simulink model "oog_example"  (R2016a)
settings: Solver=ode5  SolverMode=SingleTasking  StartTime=0.0  StopTime=Ttot  FixedStep=min(Ts_phy,Ts_sim)  RelTol=1e-3
PreLoadFcn:
  | oog_example_init
InitFcn:
  | oog_example_init
values from neighbouring files (symbols this model uses):
  col = {}    [oog_example_init.m]
  flex = {}    [oog_example_init.m]
  systemBase = {}    [oog_example_init.m]
  Ts = Ts_c    (= 0.0001)    [oog_example_init.m]
  Ts_phy = 1*Ts_sim    (= 0.0001)    [oog_example_init.m]
  Ts_sim = 100e-6    (= 0.0001)    [oog_example_init.m]
  wt1 = {}    [oog_example_init.m]
  wt2 = wt1    [oog_example_init.m]
  wt3 = wt1    [oog_example_init.m]
undefined symbols (not defined in the file or in its folder): avr, D1, Delta, DiscIntNeverNeededParam, governor, interface, Lf1, sm
libraries: powerlib x49, simulink_extras x35, pwrsysBasic x30, powerlib_meascontrol x17, pwrsysVICtrl x15, simulink x5, pwrsysVSrc x4, pwrsysTransf x4
(part 1 of 3)
settings Model: Creator=Freya_super  LastModifiedBy=ericfa
settings DataIOCC: LimitDataPoints=on  SaveFormat=Array  SaveOutput=off  SaveTime=off
settings OptimizationCC: BlockReduction=off  OptimizeBlockIOStorage=off  BufferReuse=off  GlobalBufferReuse=off  ExpressionFolding=off  LocalBlockOutputs=off
settings DebuggingCC: SolverPrmCheckMsg=warning  StateNameClashWarn=warning
settings HardwareCC: ProdBitPerPointer=32  ProdLargestAtomicFloat=None  ProdIntDivRoundTo=Undefined  ProdEndianess=Unspecified  ProdWordSize=32  ProdHWDeviceType=32-bit Generic
settings ModelReferenceCC: PropagateSignalLabelsOutOfModel=off
settings RTWCC: SystemTargetFile=rtlab_rtmodel.tlc  TemplateMakefile=rtlab_rtmodel.tmf  Description=RT-LAB Real-Time Target for Windows, and OPAL-RT Linux.
settings GRTTargetCC: GeneratePreprocessorConditionals=Use local settings  UseToolchainInfoCompliant=off
settings ConfigComp: CovModelRefEnable=Off

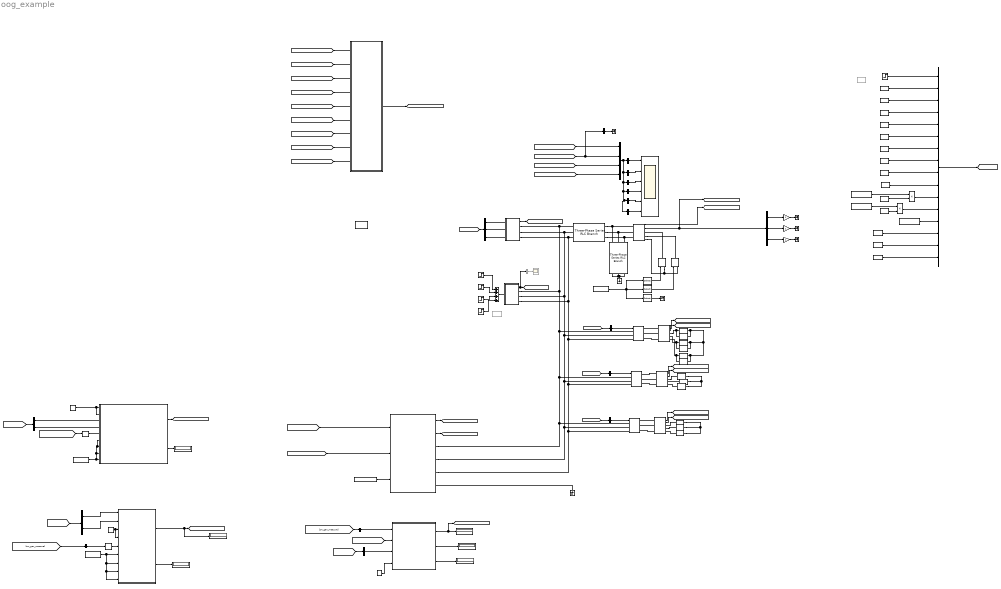
== system oog_example ==
  note: Egston terminals
  note: RMS and power calculation
  note: Automatic voltage regulator
  note: Back emf + reactance
  note: Mech.rotation
  note: Governor
  note: SM Generator (simple model)
  note: Load 3
  note: Load 2
  note: Load 1
  note: Commands
  note: Wind
      | farm
  Active : BusSelector  OutputSignals=genMeas.Pgen_pu,flexMeas.Pavg_pu,wfMeas.WT1.Pavg_pu,wfMeas.WT2.Pavg_pu,wfMeas.WT3.Pavg_pu  OutputAsBus=on
  Automatic voltage regulator : Subsystem
  Bus Creator1 : BusCreator  Inputs=4
  Bus Creator9 : BusCreator  Inputs=16
  Bus Selector1 : BusSelector  OutputSignals=load1_connect
  Bus Selector10 : BusSelector  OutputSignals=sm_backEmfPowerMeasure_pu
  Bus Selector11 : BusSelector  OutputSignals=load2_connect
  Bus Selector12 : BusSelector  OutputSignals=load3_connect
  Bus Selector4 : BusSelector  OutputSignals=freqReference pu,deltaFreqRef pu
  Bus Selector6 : BusSelector  OutputSignals=voltRef_WT1_pu,voltRef_WT2_pu,voltRef_WT3_pu
  Bus Selector7 : BusSelector  OutputSignals=freqReference pu
  Bus Selector8 : BusSelector  OutputSignals=voltRef_GT_pu,deltaVoltRef pu
  Bus Selector9 : BusSelector  OutputSignals=Vgen_filt [pu]
  Constant1 : Constant  Value=sm.phaseInitial  SampleTime=-1
  Constant{4..5,7,10,12} (5 alike) : Constant  Value=0  SampleTime=-1
  Constant13 : Constant  Commented=on  Value=0  SampleTime=Ts_sim
  Constant6 : Constant  Value=[0 0 0]  SampleTime=-1
  DC currents : BusSelector  OutputSignals=flexMeas.Idc_pu,wfMeas.WT1.Idc_pu,wfMeas.WT2.Idc_pu,wfMeas.WT3.Idc_pu  OutputAsBus=on
  DC voltages : BusSelector  OutputSignals=flexMeas.Vdc_pu,wfMeas.WT1.Vdc_pu,wfMeas.WT2.Vdc_pu,wfMeas.WT3.Vdc_pu  OutputAsBus=on
  Demux1 : Demux  Outputs=3
  Display{,1..5} (6 alike) : Display
  Flex : Subsystem
  Frequency : BusSelector  OutputSignals=genMeas.sm_freq [pu]
  Gain1 : Gain
  Gain2 : Gain
  Gain3 : Gain
  Ground1 : powerlib/Elements/Ground  LConnTagsString=a
  Ground3 : powerlib/Elements/Ground  LConnTagsString=a
  IL : powerlib/Electrical Sources/Controlled Current Source  Initialize=on  Source_Type=AC  Amplitude=0  Phase=0  Frequency=0  Measurements=None
  IL1 : powerlib/Electrical Sources/Controlled Current Source  Initialize=on  Source_Type=AC  Amplitude=0  Phase=0  Frequency=0  Measurements=None
  Memory1 : Memory
  Memory2 : Memory
  RL1 : powerlib/Elements/Series RLC Branch  LConnTagsString=__new0  RConnTagsString=__new0  BranchType=R  Resistance=load.R(1)  Inductance=load.L(1)  SetiL0=off  InitialCurrent=0  Capacitance=1e-6  Setx0=off  InitialVoltage=0  Measurements=None
  RL10 : powerlib/Elements/Series RLC Branch  LConnTagsString=__new0  RConnTagsString=__new0  BranchType=L  Resistance=load.R(1)  Inductance=load.L(1)  SetiL0=off  InitialCurrent=0  Capacitance=1e-6  Setx0=off  InitialVoltage=0  Measurements=None
  RL11 : powerlib/Elements/Series RLC Branch  LConnTagsString=__new0  RConnTagsString=__new0  BranchType=R  Resistance=load.R(1)  Inductance=load.L(1)  SetiL0=off  InitialCurrent=0  Capacitance=1e-6  Setx0=off  InitialVoltage=0  Measurements=None
  RL12 : powerlib/Elements/Series RLC Branch  LConnTagsString=__new0  RConnTagsString=__new0  BranchType=L  Resistance=load.R(1)  Inductance=load.L(1)  SetiL0=off  InitialCurrent=0  Capacitance=1e-6  Setx0=off  InitialVoltage=0  Measurements=None
  RL2 : powerlib/Elements/Series RLC Branch  LConnTagsString=__new0  RConnTagsString=__new0  BranchType=R  Resistance=load.R(1)  Inductance=load.L(1)  SetiL0=off  InitialCurrent=0  Capacitance=1e-6  Setx0=off  InitialVoltage=0  Measurements=None
  RL3 : powerlib/Elements/Series RLC Branch  LConnTagsString=__new0  RConnTagsString=__new0  BranchType=L  Resistance=load.R(1)  Inductance=load.L(1)  SetiL0=off  InitialCurrent=0  Capacitance=1e-6  Setx0=off  InitialVoltage=0  Measurements=None
  RL4 : powerlib/Elements/Series RLC Branch  LConnTagsString=__new0  RConnTagsString=__new0  BranchType=RL  Resistance=load.R(2)  Inductance=load.L(2)  SetiL0=off  InitialCurrent=0  Capacitance=1e-6  Setx0=off  InitialVoltage=0  Measurements=None
  RL5 : powerlib/Elements/Series RLC Branch  LConnTagsString=__new0  RConnTagsString=__new0  BranchType=RL  Resistance=load.R(2)  Inductance=load.L(2)  SetiL0=off  InitialCurrent=0  Capacitance=1e-6  Setx0=off  InitialVoltage=0  Measurements=None
  RL6 : powerlib/Elements/Series RLC Branch  LConnTagsString=__new0  RConnTagsString=__new0  BranchType=RL  Resistance=load.R(2)  Inductance=load.L(2)  SetiL0=off  InitialCurrent=0  Capacitance=1e-6  Setx0=off  InitialVoltage=0  Measurements=None
  RL7 : powerlib/Elements/Series RLC Branch  LConnTagsString=__new0  RConnTagsString=__new0  BranchType=RL  Resistance=load.R(3)  Inductance=load.L(3)  SetiL0=off  InitialCurrent=0  Capacitance=1e-6  Setx0=off  InitialVoltage=0  Measurements=None
  RL8 : powerlib/Elements/Series RLC Branch  LConnTagsString=__new0  RConnTagsString=__new0  BranchType=RL  Resistance=load.R(3)  Inductance=load.L(3)  SetiL0=off  InitialCurrent=0  Capacitance=1e-6  Setx0=off  InitialVoltage=0  Measurements=None
  RL9 : powerlib/Elements/Series RLC Branch  LConnTagsString=__new0  RConnTagsString=__new0  BranchType=RL  Resistance=load.R(3)  Inductance=load.L(3)  SetiL0=off  InitialCurrent=0  Capacitance=1e-6  Setx0=off  InitialVoltage=0  Measurements=None
  Reactive : BusSelector  OutputSignals=genMeas.Qgen_pu,flexMeas.Qavg_pu,wfMeas.WT1.Qavg_pu,wfMeas.WT2.Qavg_pu,wfMeas.WT3.Qavg_pu  OutputAsBus=on
  Rotation1 : Subsystem
  SM_simple : Subsystem
  Scope_All : Scope  NumInputPorts=6
  Scope_Flex : Scope  Commented=on
  Selector6 : Selector  InputPortWidth=3  IndexOptions=Index vector (dialog)  Indices=[1]  OutputSizes=1
  Selector7 : Selector  InputPortWidth=3  IndexOptions=Index vector (dialog)  Indices=2  OutputSizes=1
  Selector8 : Selector  InputPortWidth=3  IndexOptions=Index vector (dialog)  Indices=3  OutputSizes=1
  Step : Step  Time=3  SampleTime=0
  Step1 : Step  Time=7  After=-0.2  SampleTime=0
  Step2 : Step  Time=7.5  After=-0.2  SampleTime=0
  Step3 : Step  Time=8  After=-0.2  SampleTime=0
  Step4 : Step  Time=8.5  After=-0.2  SampleTime=0
  Sum : Sum  Inputs=4
  Terminator{,1..4} (5 alike) : Terminator
  Three-Phase Series RLC Branch : powerlib/Elements/Three-Phase Series RLC Branch  LConnTagsString=A|B|C  RConnTagsString=A|B|C  BranchType=R  Resistance=interface.Rs  Inductance=1e-3  Capacitance=1e-6  Measurements=None
  Three-Phase Series RLC Branch1 : powerlib/Elements/Three-Phase Series RLC Branch  LConnTagsString=A|B|C  RConnTagsString=A|B|C  BranchType=R  Resistance=interface.Rp  Inductance=1e-3  Capacitance=1e-6  Measurements=None
  Three-Phase V-I Measurement{,1..3} (4 alike) : powerlib/Measurements/Three-Phase V-I Measurement  VoltageMeasurement=phase-to-ground  SetLabelV=off  LabelV=Vabc  Vpu=off  VpuLL=off  CurrentMeasurement=yes  SetLabelI=off  LabelI=Iabc  Ipu=off  Pbase=100e6  Vbase=500e3  OutputType=Complex  PhasorSimulation=off  PSBequivalent=0
  Three-Phase Breaker : powerlib/Elements/Three-Phase Breaker  InitialState=open  SwitchA=on  SwitchB=on  SwitchC=on  SwitchTimes="[4/60  10/60]"  External=on  BreakerResistance=0.001  SnubberResistance=1e6  SnubberCapacitance=inf  Measurements=None
  Three-Phase Breaker1 : powerlib/Elements/Three-Phase Breaker  InitialState=open  SwitchA=on  SwitchB=on  SwitchC=on  SwitchTimes="[4/60  10/60]"  External=on  BreakerResistance=0.001  SnubberResistance=1e6  SnubberCapacitance=inf  Measurements=None
  Three-Phase Breaker2 : powerlib/Elements/Three-Phase Breaker  InitialState=open  SwitchA=on  SwitchB=on  SwitchC=on  SwitchTimes="[4/60  10/60]"  External=on  BreakerResistance=0.001  SnubberResistance=1e6  SnubberCapacitance=inf  Measurements=None
  Trigger_Data_Logging : Constant  Value=0  SampleTime=-1
  Turbine Governor1 : Subsystem
  Voltage : BusSelector  OutputSignals=genMeas.Vgen_filt [pu],flexMeas.Vavg_pu,wfMeas.WT1.Vavg_pu,wfMeas.WT2.Vavg_pu,wfMeas.WT3.Vavg_pu  OutputAsBus=on
  Wind Farm : Subsystem
  current_gain : Constant  Value=0.1  SampleTime=-1
  deltaFreqRef pu : Constant  Value=0  OutDataTypeStr=double  SampleTime=Ts
  deltaVoltRef pu : Constant  Value=0  OutDataTypeStr=double  SampleTime=Ts
  dfreqRefESS : Constant  Value=0  OutDataTypeStr=double  SampleTime=Ts
  dfreqRefGT : Constant  Value=0  OutDataTypeStr=double  SampleTime=Ts
  enableCurrentFeedback : Constant  Value=0  OutDataTypeStr=double  SampleTime=Ts
  enableVoltageOutput : Constant  Value=0  OutDataTypeStr=double  SampleTime=Ts
  flex : BusSelector  Commented=on  OutputSignals=Pavg_pu,Qavg_pu,Vavg_pu,Vdc_pu,Idc_pu  OutputAsBus=on
  freqReference pu : Constant  OutDataTypeStr=double  SampleTime=Ts
  gen : BusSelector  OutputSignals=Pgen_pu,Qgen_pu,Vgen_filt [pu]  OutputAsBus=on
  load1_connect : Constant  Commented=on  Value=0  OutDataTypeStr=double  SampleTime=Ts
  load2_connect : Constant  Value=0  OutDataTypeStr=double  SampleTime=Ts
  load3_connect : Constant  Value=0  OutDataTypeStr=double  SampleTime=Ts
  mul : Product  Inputs=**
  mul1 : Product  Inputs=**
  powergui : powerlib/powergui  Priority=1  SimulationMode=Discrete  SolverType=Tustin  SampleTime=max(Ts_phy,Ts_sim)  frequency=60  SPID=off  DisableSnubberDevices=off  DisableRonSwitches=off  DisableVfSwitches=off  SwTol=0  DisplayEquations=off  Interpol=off  ExternalGateDelay=off  methode=off  Ts=0  FunctionMessages=off  echomessages=off  HookPort=off  EnableUseOfTLC=off  x0status=blocks  frequencyindice=0  Pbase=100e6  ErrMax=1e-4  Iterations=50  UnitsV=kV  UnitsW=MW  buscounter=0  RestoreLinks=warning  ResistiveCurrentMeasurement=off  Frange=[0:2:500]  Ylog=off  Xlog=on  ShowGrid=off  save=off  variable=ZData  structure=0  ZoomFFT=off  StartTime=0.0  cycles=1  DisplayStyle=1  fundamental=60  FreqAxis=off  MaxFrequency=1000  frequencyindicesteady=1  RmsSteady=1  display=off
  rms and power calc : Subsystem
  voltRefESS : Constant  OutDataTypeStr=double  SampleTime=Ts
  voltRefGT : Constant  OutDataTypeStr=double  SampleTime=Ts
  voltRefWT1 : Constant  OutDataTypeStr=double  SampleTime=Ts
  voltRefWT2 : Constant  OutDataTypeStr=double  SampleTime=Ts
  voltRefWT3 : Constant  OutDataTypeStr=double  SampleTime=Ts
  voltage_gain : Constant  Value=0.1  SampleTime=-1
  wires:
  Bus Selector12/1 -> Three-Phase Breaker2/1  "<load3_connect>"
  [fromGUI] -> Bus Selector12/1
  Bus Selector11/1 -> Three-Phase Breaker1/1  "<load2_connect>"
  [fromGUI] -> Bus Selector11/1
  Bus Selector1/1 -> Three-Phase Breaker/1  "<load1_connect>"
  [fromGUI] -> Bus Selector1/1
  Three-Phase V-I Measurement2/1 -> [V_abc_L3]
  Three-Phase V-I Measurement2/2 -> [I_abc_L3]
  Three-Phase V-I Measurement1/1 -> [V_abc_L2]
  Three-Phase V-I Measurement1/2 -> [I_abc_L2]
  Three-Phase V-I Measurement3/2 -> [I_abc_L1]
  Three-Phase V-I Measurement3/1 -> [V_abc_L1]
  Bus Selector10/1 -> Rotation1/1(generator power (pu))  "<sm_backEmfPowerMeasure_pu>"
  [sm_gen_measure] -> Bus Selector10/1
  Bus Selector9/1 -> Memory2/1  "<Vgen_filt [pu]>"
  SM_simple/1(wt1) -> [wt]
  Memory2/1 -> Automatic voltage regulator/5(voltage_feedback (pu))
  Constant7/1 -> Rotation1/4(resetSpeed)
  Constant12/1 -> Automatic voltage regulator/6(qGen (pu)), Automatic voltage regulator/7(qRefDroop (pu)), Automatic voltage regulator/8(pGen (pu)), Automatic voltage regulator/9(pRefDroop (pu))
  Constant4/1 -> Automatic voltage regulator/4(Reset_integrator), Automatic voltage regulator/3(Reset_value)
  Bus Selector8/2 -> Automatic voltage regulator/2(deltaVoltageRef (pu))  "<deltaVoltRef pu>"
  Constant10/1 -> Turbine Governor1/9(pGen (pu)), Turbine Governor1/8(powerControlEnable), Turbine Governor1/7(pRef (pu)), Turbine Governor1/6(pRefDroop (pu))
  Bus Selector4/2 -> Turbine Governor1/4(deltaSpeedRef (pu))  "<deltaFreqRef pu>"
  Bus Selector4/1 -> Turbine Governor1/3(Speed_ref (pu))  "<freqReference pu>"
  Constant5/1 -> Turbine Governor1/2(Reset_value), Turbine Governor1/1(Reset_gov)  "<resetSpeedGov>"
  Bus Selector8/1 -> Automatic voltage regulator/1(Voltage_ref (pu))  "<voltRef_GT_pu>"
  [fromGUI] -> Bus Selector8/1
  Bus Selector7/1 -> Rotation1/3(InitialSpeed)  "<freqReference pu>"
  [fromGUI] -> Bus Selector7/1
  [fromGUI] -> Bus Selector4/1
  [drivingTorque_pu] -> Rotation1/2(driving torque (pu))
  Turbine Governor1/1(output (pu)) -> [drivingTorque_pu]
  [sm_gen_measure] -> Bus Selector9/1
  Automatic voltage regulator/2(voltageRefActual (pu)) -> Display5/1
  Automatic voltage regulator/1(output (pu)) -> Display3/1, [sm_dynamicVoltage_pu]
  Turbine Governor1/2(speedRefActual (pu)) -> Display4/1
  Memory1/1 -> Turbine Governor1/5(Speed_feedback (pu))
  [sm_dynamicSpeed_pu] -> Memory1/1
  Rotation1/3(electric torque (pu)) -> Display2/1
  Rotation1/2(mechanical torque (pu)) -> Display1/1
  Rotation1/1(turbine speed (pu)) -> Display/1, [sm_dynamicSpeed_pu]
  [sm_dynamicVoltage_pu] -> SM_simple/2(GenBackEmf [pu])
  SM_simple/2(sm_gen_measure) -> [sm_gen_measure]
  Constant1/1 -> SM_simple/3(Phase [rad])
  [sm_dynamicSpeed_pu] -> SM_simple/1(Frequency [pu])  "sm_freq"
  Gain3/1 -> Terminator3/1  "Ic"
  Demux1/3 -> Gain3/1
  Gain2/1 -> Terminator2/1  "Ib"
  Demux1/2 -> Gain2/1
  Gain1/1 -> Terminator1/1  "Ia"
  Demux1/1 -> Gain1/1
  Selector7/1 -> IL1/1
  Three-Phase V-I Measurement/2 -> Demux1/1, [I_abc_interface]  "I_abc"
  Selector8/1 -> Terminator/1
  Constant6/1 -> Selector6/1, Selector7/1, Selector8/1
  Three-Phase V-I Measurement/1 -> [V_abc_interface]  "V_abc"
  Selector6/1 -> IL/1
  [wt] -> rms and power calc/1(wt)
  [V_abc_L1] -> rms and power calc/2(L1_Vabc)
  [I_abc_L1] -> rms and power calc/3(L1_Iabc)
  [V_abc_L2] -> rms and power calc/4(L2_Vabc)
  [I_abc_L2] -> rms and power calc/5(L2_Iabc)
  [V_abc_L3] -> rms and power calc/6(L3_Vabc)
  [I_abc_L3] -> rms and power calc/7(L3_Iabc)
  [V_abc_interface] -> rms and power calc/8(Interface_Vabc)
  [I_abc_interface] -> rms and power calc/9(Interface_Iabc)
  rms and power calc/1(Out1) -> [electricModel_meas]
  deltaVoltRef pu/1 -> Bus Creator9/15  "deltaVoltRef pu"
  dfreqRefGT/1 -> Bus Creator9/9  "dfreqRef_GT_pu"
  deltaFreqRef pu/1 -> Bus Creator9/14  "deltaFreqRef pu"
  dfreqRefESS/1 -> Bus Creator9/10  "dfreqRef_ESS_pu"
  voltage_gain/1 -> mul1/1  "voltage_gain_grid_side"
  mul1/1 -> Bus Creator9/12  "voltage_gain_grid_side"
  voltRefESS/1 -> Bus Creator9/5  "voltRef_ESS_pu"
  voltRefWT1/1 -> Bus Creator9/6  "voltRef_WT1_pu"
  current_gain/1 -> mul/1  "PHIL_gain_grid_side"
  Bus Creator9/1 -> [fromGUI]  "fromGUI"
  voltRefWT3/1 -> Bus Creator9/8  "voltRef_WT3_pu"
  Trigger_Data_Logging/1 -> Bus Creator9/13  "enable_logging"
  load2_connect/1 -> Bus Creator9/2  "load2_connect"
  mul/1 -> Bus Creator9/11  "PHIL_gain_grid_side"
  voltRefWT2/1 -> Bus Creator9/7  "voltRef_WT2_pu"
  enableCurrentFeedback/1 -> mul/2
  Step/1 -> Bus Creator9/1  "load1_connect"
  load3_connect/1 -> Bus Creator9/3  "load3_connect"
  enableVoltageOutput/1 -> mul1/2
  voltRefGT/1 -> Bus Creator9/4  "voltRef_GT_pu"
  [wf_measure] -> Bus Creator1/4  "wfMeas"
  [electricModel_meas] -> Bus Creator1/1  "electricModel_meas"
  [sm_gen_measure] -> gen/1, Bus Creator1/2  "genMeas"
  [flex_measure] -> Bus Creator1/3  "flexMeas"
  freqReference pu/1 -> Bus Creator9/16  "freqReference pu"
  Voltage/1 -> Scope_All/1
  Reactive/1 -> Scope_All/2
  Frequency/1 -> Scope_All/3  "<sm_freq [pu]>"
  Active/1 -> Scope_All/4
  Wind Farm/1(m) -> [wf_measure]  "WF"
  Bus Selector6/2 -> Wind Farm/2(WT2_Vsp)  "<voltRef_WT2_pu>"
  Bus Selector6/3 -> Wind Farm/3(WT1_Vsp)  "<voltRef_WT3_pu>"
  Bus Selector6/1 -> Wind Farm/1(WT3_Vsp)  "<voltRef_WT1_pu>"
  [fromGUI] -> Bus Selector6/1
  Bus Creator1/1 -> Voltage/1, Reactive/1, DC currents/1, DC voltages/1, Active/1, Frequency/1
  Flex/1(m) -> flex/1, [flex_measure]
  flex/1 -> Scope_Flex/1
  Sum/1 -> Flex/1(Psp)
  Step1/1 -> Sum/1
  Step2/1 -> Sum/2
  Step3/1 -> Sum/3
  gen/1 -> Terminator4/1
  DC voltages/1 -> Scope_All/5
  DC currents/1 -> Scope_All/6
  Step4/1 -> Sum/4
  connections:
  RL9/RConn1 -- RL7/RConn1 -- RL8/RConn1
  RL4/RConn1 -- RL5/RConn1 -- RL6/RConn1
  RL1/RConn1 -- RL10/RConn1 -- RL12/RConn1 -- RL11/RConn1 -- RL3/RConn1 -- RL2/RConn1
  Three-Phase Breaker/LConn3 -- Three-Phase Breaker1/LConn3 -- Three-Phase Breaker2/LConn3 -- SM_simple/RConn3 -- Flex/RConn3 -- Wind Farm/RConn3 -- Three-Phase Series RLC Branch/LConn3
  Three-Phase Series RLC Branch/RConn1 -- Three-Phase V-I Measurement/LConn1 -- Three-Phase Series RLC Branch1/RConn1
  Three-Phase Series RLC Branch/RConn2 -- Three-Phase V-I Measurement/LConn2 -- Three-Phase Series RLC Branch1/RConn2
  Three-Phase Series RLC Branch/RConn3 -- Three-Phase V-I Measurement/LConn3 -- Three-Phase Series RLC Branch1/RConn3
  Three-Phase Series RLC Branch1/LConn1 -- Three-Phase Series RLC Branch1/LConn3 -- Ground1/LConn1 -- Three-Phase Series RLC Branch1/LConn2
  IL/LConn1 -- Three-Phase V-I Measurement/RConn3 -- IL1/LConn1
  Three-Phase V-I Measurement3/LConn1 -- Three-Phase Breaker/RConn1
  Three-Phase V-I Measurement3/RConn1 -- RL10/LConn1 -- RL1/LConn1
  Three-Phase V-I Measurement2/LConn3 -- Three-Phase Breaker2/RConn3
  Ground3/LConn1 -- SM_simple/RConn4
  Three-Phase V-I Measurement2/RConn2 -- RL9/LConn1
  Three-Phase V-I Measurement3/LConn2 -- Three-Phase Breaker/RConn2
  Three-Phase V-I Measurement1/LConn1 -- Three-Phase Breaker1/RConn1
  RL7/LConn1 -- Three-Phase V-I Measurement2/RConn3
  RL6/LConn1 -- Three-Phase V-I Measurement1/RConn3
  Three-Phase V-I Measurement1/RConn1 -- RL4/LConn1
  RL8/LConn1 -- Three-Phase V-I Measurement2/RConn1
  Three-Phase V-I Measurement2/LConn2 -- Three-Phase Breaker2/RConn2
  Three-Phase V-I Measurement1/LConn2 -- Three-Phase Breaker1/RConn2
  RL11/LConn1 -- RL12/LConn1 -- Three-Phase V-I Measurement3/RConn3
  Three-Phase V-I Measurement1/LConn3 -- Three-Phase Breaker1/RConn3
  Three-Phase V-I Measurement/RConn2 -- IL1/RConn1
  Three-Phase V-I Measurement2/LConn1 -- Three-Phase Breaker2/RConn1
  IL/RConn1 -- Three-Phase V-I Measurement/RConn1
  Three-Phase V-I Measurement3/LConn3 -- Three-Phase Breaker/RConn3
  RL2/LConn1 -- RL3/LConn1 -- Three-Phase V-I Measurement3/RConn2
  RL5/LConn1 -- Three-Phase V-I Measurement1/RConn2
  Three-Phase Breaker1/LConn2 -- Three-Phase Breaker2/LConn2 -- SM_simple/RConn2 -- Three-Phase Breaker/LConn2 -- Flex/RConn2 -- Wind Farm/RConn2 -- Three-Phase Series RLC Branch/LConn2
  Three-Phase Breaker/LConn1 -- Three-Phase Breaker1/LConn1 -- Three-Phase Breaker2/LConn1 -- SM_simple/RConn1 -- Flex/RConn1 -- Wind Farm/RConn1 -- Three-Phase Series RLC Branch/LConn1

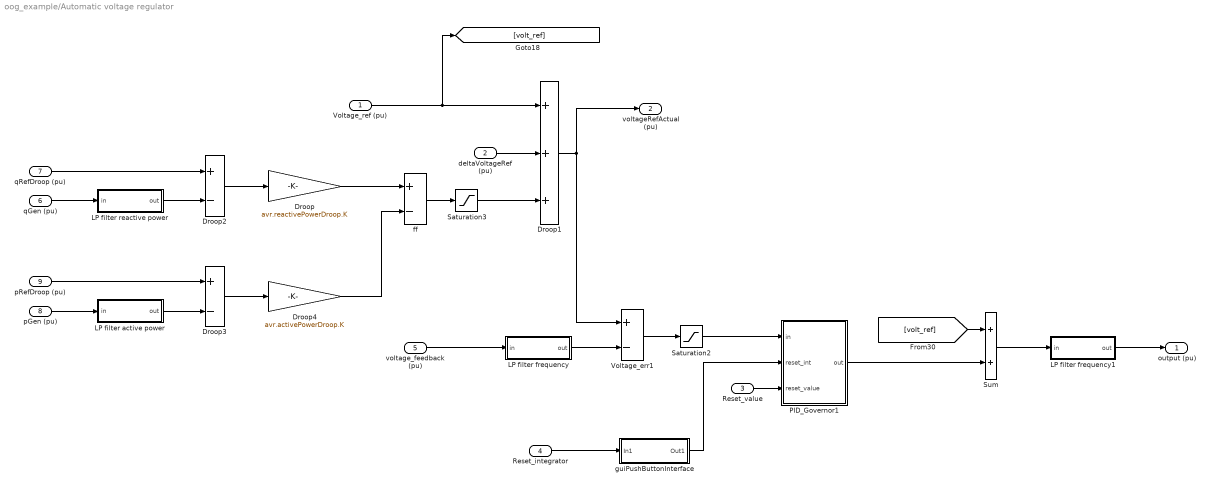
== system oog_example/Automatic voltage regulator ==
  Voltage_ref (pu) : Inport
  deltaVoltageRef (pu) : Inport  Port=2
  Reset_value : Inport  Port=3
  Reset_integrator : Inport  Port=4
  voltage_feedback (pu) : Inport  Port=5
  qGen (pu) : Inport  Port=6
  qRefDroop (pu) : Inport  Port=7
  pGen (pu) : Inport  Port=8
  pRefDroop (pu) : Inport  Port=9
  Droop : Gain  Gain=avr.reactivePowerDroop.K
  Droop1 : Sum  Inputs=+++
  Droop2 : Sum  Inputs=+-
  Droop3 : Sum  Inputs=+-
  Droop4 : Gain  Gain=avr.activePowerDroop.K
  LP filter active power : Subsystem  mask(Discrete first order low pass filter){tau=avr.LPfilterPowerMeasurementDroop.T, Ts=Ts, x0=0, y0=0}
      mask prompts: tau "Filter time constant [s]"; Ts "Sampling time [s]"; x0 "Initial input"; y0 "Initial output"
      mask help: Discrete first order low pass filter derived from a continous filter by bilinear transformation.
  LP filter frequency : Subsystem  mask(Discrete first order low pass filter){tau=avr.LPfilterVoltageMeasurement.T, Ts=Ts, x0=0, y0=0}
      mask prompts: tau "Filter time constant [s]"; Ts "Sampling time [s]"; x0 "Initial input"; y0 "Initial output"
      mask help: Discrete first order low pass filter derived from a continous filter by bilinear transformation.
  LP filter frequency1 : Subsystem  mask(Discrete first order low pass filter){tau=avr.fieldWinding.T, Ts=Ts, x0=avr.init, y0=avr.init}
      mask prompts: tau "Filter time constant [s]"; Ts "Sampling time [s]"; x0 "Initial input"; y0 "Initial output"
      mask help: Discrete first order low pass filter derived from a continous filter by bilinear transformation.
  LP filter reactive power : Subsystem  mask(Discrete first order low pass filter){tau=avr.LPfilterReactivePowerMeasurementDroop.T, Ts=Ts, x0=0, y0=0}
      mask prompts: tau "Filter time constant [s]"; Ts "Sampling time [s]"; x0 "Initial input"; y0 "Initial output"
      mask help: Discrete first order low pass filter derived from a continous filter by bilinear transformation.
  PID_Governor1 : Subsystem  mask(Discrete PI with parallel form){kp=avr.kP, ki=avr.kI, kd=avr.kd, Tlp=avr.derivativeLP, xi=0, up_sat_limit=avr.saturationUpper, low_sat_limit=avr.saturationLower}
      mask prompts: kp "Proportional gain"; ki "Integral gain"; kd "Derivative gain"; Tlp "Derivative LP filter T"; xi "Initial condition integrator"; up_sat_limit "Saturation upper limit"; low_sat_limit "Saturation lower limit"
      mask help: Discrete PI in parallel form with saturation on the integrator and on the output. The upper and the lower saturation limits are fixed.
  Saturation2 : Saturate  UpperLimit=avr.ErrMax  LowerLimit=avr.ErrMin
  Saturation3 : Saturate  UpperLimit=avr.droopSaturationUpper  LowerLimit=avr.droopSaturationLower
  Sum : Sum
  Voltage_err1 : Sum  Inputs=+-
  ff : Sum  Inputs=+-
  guiPushButtonInterface : Subsystem
  output (pu) : Outport
  voltageRefActual (pu) : Outport  Port=2
  wires:
  guiPushButtonInterface/1(Out1) -> PID_Governor1/2(reset_int)
  Reset_value/1 -> PID_Governor1/3(reset_value)
  Sum/1 -> LP filter frequency1/1(in)
  [volt_ref] -> Sum/1
  ff/1 -> Saturation3/1
  Droop4/1 -> ff/2
  Droop3/1 -> Droop4/1
  LP filter active power/1(out) -> Droop3/2
  pRefDroop (pu)/1 -> Droop3/1
  pGen (pu)/1 -> LP filter active power/1(in)
  LP filter frequency1/1(out) -> output (pu)/1
  Saturation3/1 -> Droop1/3
  Saturation2/1 -> PID_Governor1/1(in)
  deltaVoltageRef (pu)/1 -> Droop1/2
  Droop2/1 -> Droop/1
  LP filter reactive power/1(out) -> Droop2/2
  qRefDroop (pu)/1 -> Droop2/1
  qGen (pu)/1 -> LP filter reactive power/1(in)
  Voltage_err1/1 -> Saturation2/1
  Droop/1 -> ff/1
  LP filter frequency/1(out) -> Voltage_err1/2
  PID_Governor1/1(out) -> Sum/2
  Reset_integrator/1 -> guiPushButtonInterface/1(In1)
  Droop1/1 -> voltageRefActual (pu)/1, Voltage_err1/1
  voltage_feedback (pu)/1 -> LP filter frequency/1(in)
  Voltage_ref (pu)/1 -> Droop1/1, [volt_ref]

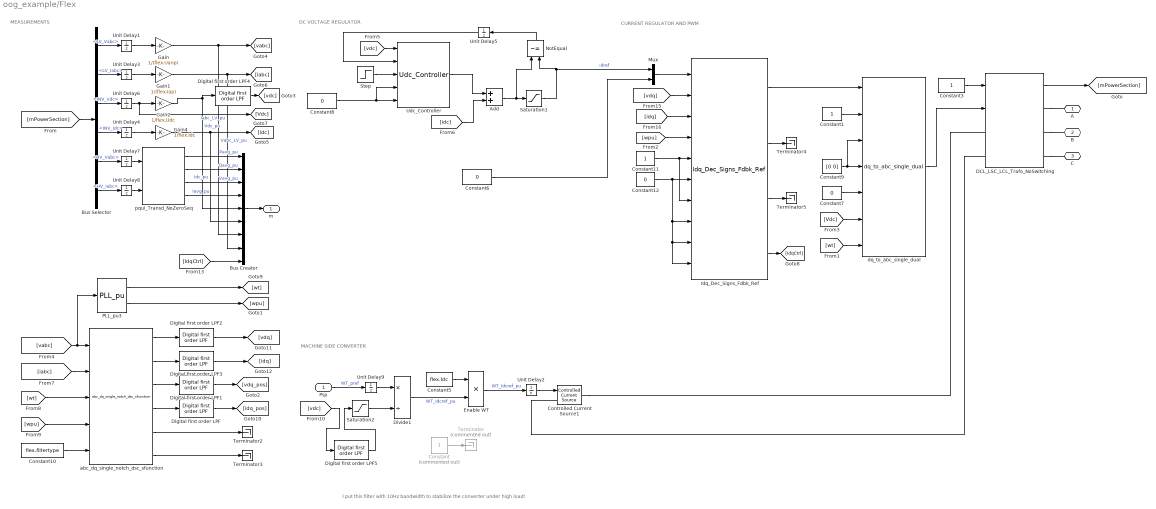
== system oog_example/Flex ==
  note: I put this filter with 10Hz bandwidth to stabilize the converter under high load!
  note: MEASUREMENTS
  note: MACHINE SIDE CONVERTER
  note: DC VOLTAGE REGULATOR
  note: CURRENT REGULATOR AND PWM
  Psp : Inport
  Add : Sum
  Bus Creator : BusCreator  Inputs=9
  Bus Selector : BusSelector  OutputSignals=LV_Vabc,LV_Iabc,INV_Vdc,INV_Idc,HV_Vabc,HV_Iabc
  Constant : Constant  Commented=on
  Constant1 : Constant  SampleTime=flex.Ts_control
  Constant10 : Constant  Value=flex.filtertype  SampleTime=flex.Ts_control
  Constant11 : Constant  SampleTime=flex.Ts_control
  Constant{6..8,12} (4 alike) : Constant  Value=0  SampleTime=flex.Ts_control
  Constant3 : Constant  SampleTime=flex.Ts_control
  Constant5 : Constant  Value=flex.Idc  SampleTime=flex.Ts_control
  Constant9 : Constant  Value=[0 0]  SampleTime=flex.Ts_control
  Controlled Current Source1 : powerlib/Electrical Sources/Controlled Current Source  Initialize=on  Source_Type=DC  Amplitude=0  Phase=0  Frequency=50  Measurements=None
  DCL_LSC_LCL_Trafo_NoSwitching : pwrsysVSrc/DCL_LSC_LCL_Trafo_NoSwitching  Sn=flex.Sn  fn=systemBase.fn  Uhv_ab=systemBase.Vn  Uab=flex.Un  lf2=flex.LCL.l2  rf2=flex.LCL.r2  Lf1=flex.LCL.L1  Rf1=flex.LCL.R1  Cf=flex.LCL.Cf  Rc=flex.LCL.Rf  Cdc=flex.Cdc  Udc0=flex.Udc  Tsm=flex.Ts_control  Tstart=flex.DCVCont.Start
  Digital first order LPF : pwrsysBasic/Digital first order LPF  Ts=wt1.Ts_control  fcutout=wt1.CurrCont.f_LPF_noise
  Digital first order LPF1 : pwrsysBasic/Digital first order LPF  Ts=flex.Ts_control  fcutout=flex.CurrCont.f_LPF_noise
  Digital first order LPF2 : pwrsysBasic/Digital first order LPF  Ts=flex.Ts_control  fcutout=flex.CurrCont.f_LPF_noise
  Digital first order LPF3 : pwrsysBasic/Digital first order LPF  Ts=wt1.Ts_control  fcutout=wt1.CurrCont.f_LPF_noise
  Digital first order LPF4 : pwrsysBasic/Digital first order LPF  Ts=flex.Ts_control  fcutout=flex.CurrCont.f_LPF_noise
  Digital first order LPF5 : pwrsysBasic/Digital first order LPF  Ts=flex.Ts_control  fcutout=10
  Divide1 : Product  Inputs=*/
  Enable WT : Product  Inputs=**
  Gain : Gain  Gain=1/(flex.Uanp)
  Gain1 : Gain  Gain=1/(flex.Iap)
  Gain2 : Gain  Gain=1/flex.Udc
  Gain4 : Gain  Gain=1/flex.Idc
  Idq_Dec_Signs_Fdbk_Ref : pwrsysVICtrl/Idq_Dec_Signs_Fdbk_Ref  Ts=flex.Ts_control  fn=systemBase.fn  Kp=flex.CurrContSingle.kp  Ti=flex.CurrContSingle.Ti  L=flex.CurrCont.x  PI_max=flex.CurrCont.PImax  PI_min=flex.CurrCont.PImin  TrafoPhaseComp=0
  Mux : Mux  Inputs=2
  NotEqual : RelationalOperator  Operator=~=  OutDataTypeStr=boolean
  PLL_pu3 : pwrsysBasic/PLL_pu  fn=systemBase.fn  Ts=flex.Ts_control  Kp_pll=90  Ki_pll=1200  Kd_pll=0  PLL_ini=60
  Saturation1 : Saturate  UpperLimit=flex.DCVCont.PImax  LowerLimit=flex.DCVCont.PImin
  Saturation2 : Saturate  UpperLimit=1.2  LowerLimit=0.8
  Step : Step  Time=flex.DCVCont.Start  SampleTime=0
  Terminator : Terminator  Commented=on
  Terminator{2..5} (4 alike) : Terminator
  Udc_Controller : pwrsysVICtrl/Udc_Controller  Ts=flex.Ts_control  Kp=flex.DCVContSingle.kp  Ti=flex.DCVContSingle.Ti  PI_max=flex.DCVCont.PImax  PI_min=flex.DCVCont.PImin
  Unit Delay{1,3,7..8} (4 alike) : UnitDelay  InitialCondition=[0 0 0]  SampleTime=flex.Ts_control
  Unit Delay{2,4..5,9} (4 alike) : UnitDelay  SampleTime=flex.Ts_control
  Unit Delay6 : UnitDelay  InitialCondition=1  SampleTime=flex.Ts_control
  abc_dq_single_notch_dsc_sfunction : pwrsysTransf/abc_dq_single_notch_dsc_sfunction  Ts=flex.Ts_control  fn=2*systemBase.fn  zeta=flex.CurrCont.zeta
  dq_to_abc_single_dual : pwrsysVICtrl/dq_to_abc_single_dual  Ts=flex.Ts_control  Uabp=flex.Uabp
  pqui_Transd_NoZeroSeq : pwrsysBasic/pqui_Transd_NoZeroSeq  Sn=flex.Sn  Uanp=systemBase.Vn*(2/3)^0.5  Iap=flex.Iap*(flex.Un/systemBase.Vn)
  A : PMIOPort  Port=1  Side=Right
  B : PMIOPort  Port=2  Side=Right
  C : PMIOPort  Port=3  Side=Right
  m : Outport
  wires:
  Divide1/1 -> Enable WT/2  "WT_Idcref_pu"
  Bus Selector/1 -> Unit Delay1/1  "<LV_Vabc>"
  Unit Delay2/1 -> Controlled Current Source1/1
  Gain1/1 -> Bus Creator/8, [iabc]  "Iabc_LV_pu"
  Bus Selector/2 -> Unit Delay3/1  "<LV_Iabc>"
  Constant6/1 -> Mux/2
  Constant5/1 -> Enable WT/1
  [mPowerSection] -> Bus Selector/1
  Enable WT/1 -> Unit Delay2/1  "WT_Idcref_pu"
  Gain/1 -> Bus Creator/7, [vabc]  "Vabc_LV_pu"
  Constant8/1 -> Udc_Controller/4, Udc_Controller/5
  NotEqual/1 -> Unit Delay5/1
  [vdc] -> Udc_Controller/1
  Unit Delay5/1 -> Udc_Controller/2
  Saturation1/1 -> NotEqual/2, Mux/1  "idref"
  [idc] -> Add/2
  Udc_Controller/1 -> Add/1
  Add/1 -> NotEqual/1, Saturation1/1
  Step/1 -> Udc_Controller/3
  [idq] -> Idq_Dec_Signs_Fdbk_Ref/3
  [Vdc] -> dq_to_abc_single_dual/6
  [wpu] -> Idq_Dec_Signs_Fdbk_Ref/4
  dq_to_abc_single_dual/1 -> DCL_LSC_LCL_Trafo_NoSwitching/2
  Mux/1 -> Idq_Dec_Signs_Fdbk_Ref/1
  Constant3/1 -> DCL_LSC_LCL_Trafo_NoSwitching/1
  Psp/1 -> Unit Delay9/1  "WT_pref"
  [vdc] -> Digital first order LPF5/1
  [wt] -> dq_to_abc_single_dual/7
  Constant10/1 -> abc_dq_single_notch_dsc_sfunction/5
  Bus Selector/5 -> Unit Delay7/1  "<HV_Vabc>"
  Bus Selector/6 -> Unit Delay8/1  "<HV_Iabc>"
  pqui_Transd_NoZeroSeq/1 -> Bus Creator/1  "Pavg_pu"
  pqui_Transd_NoZeroSeq/2 -> Bus Creator/2  "Qavg_pu"
  pqui_Transd_NoZeroSeq/3 -> Bus Creator/3  "Vavg_pu"
  pqui_Transd_NoZeroSeq/4 -> Bus Creator/4  "Iavg_pu"
  Bus Creator/1 -> m/1
  Bus Selector/3 -> Unit Delay6/1  "<INV_Vdc>"
  Gain2/1 -> Bus Creator/5, Digital first order LPF4/1  "Vdc_pu"
  Gain4/1 -> [idc], Bus Creator/6  "Idc_pu"
  Bus Selector/4 -> Unit Delay4/1  "<INV_Idc>"
  PLL_pu3/2 -> [wpu]
  PLL_pu3/1 -> [wt]
  DCL_LSC_LCL_Trafo_NoSwitching/1 -> [mPowerSection]
  Unit Delay1/1 -> Gain/1
  Unit Delay3/1 -> Gain1/1
  Unit Delay4/1 -> Gain4/1
  Unit Delay8/1 -> pqui_Transd_NoZeroSeq/2
  Unit Delay6/1 -> [Vdc], Gain2/1
  Unit Delay7/1 -> pqui_Transd_NoZeroSeq/1
  Unit Delay9/1 -> Divide1/1
  abc_dq_single_notch_dsc_sfunction/6 -> Terminator3/1
  abc_dq_single_notch_dsc_sfunction/5 -> Terminator2/1
  Idq_Dec_Signs_Fdbk_Ref/2 -> Terminator4/1
  [vdq] -> Idq_Dec_Signs_Fdbk_Ref/2
  Constant1/1 -> dq_to_abc_single_dual/2
  Constant7/1 -> dq_to_abc_single_dual/5
  Constant9/1 -> dq_to_abc_single_dual/4, dq_to_abc_single_dual/3
  Constant11/1 -> Idq_Dec_Signs_Fdbk_Ref/7, Idq_Dec_Signs_Fdbk_Ref/5
  Constant12/1 -> Idq_Dec_Signs_Fdbk_Ref/8, Idq_Dec_Signs_Fdbk_Ref/9, Idq_Dec_Signs_Fdbk_Ref/10, Idq_Dec_Signs_Fdbk_Ref/6
  Idq_Dec_Signs_Fdbk_Ref/3 -> Terminator5/1
  Idq_Dec_Signs_Fdbk_Ref/4 -> [IdqCtrl]
  [IdqCtrl] -> Bus Creator/9
  Idq_Dec_Signs_Fdbk_Ref/1 -> dq_to_abc_single_dual/1
  [wt] -> abc_dq_single_notch_dsc_sfunction/3
  [wpu] -> abc_dq_single_notch_dsc_sfunction/4
  abc_dq_single_notch_dsc_sfunction/1 -> Digital first order LPF2/1
  [vabc] -> abc_dq_single_notch_dsc_sfunction/1, PLL_pu3/1
  [iabc] -> abc_dq_single_notch_dsc_sfunction/2
  abc_dq_single_notch_dsc_sfunction/3 -> Digital first order LPF1/1
  abc_dq_single_notch_dsc_sfunction/4 -> Digital first order LPF/1
  abc_dq_single_notch_dsc_sfunction/2 -> Digital first order LPF3/1
  Digital first order LPF/1 -> [idq_pos]
  Digital first order LPF1/1 -> [vdq_pos]
  Digital first order LPF2/1 -> [vdq]
  Digital first order LPF3/1 -> [idq]
  Digital first order LPF4/1 -> [vdc]
  Constant/1 -> Terminator/1
  Saturation2/1 -> Divide1/2
  Digital first order LPF5/1 -> Saturation2/1
  connections:
  Controlled Current Source1/RConn1 -- DCL_LSC_LCL_Trafo_NoSwitching/LConn1
  DCL_LSC_LCL_Trafo_NoSwitching/RConn3 -- C/RConn1
  DCL_LSC_LCL_Trafo_NoSwitching/RConn1 -- A/RConn1
  DCL_LSC_LCL_Trafo_NoSwitching/RConn2 -- B/RConn1
  Controlled Current Source1/LConn1 -- DCL_LSC_LCL_Trafo_NoSwitching/LConn2

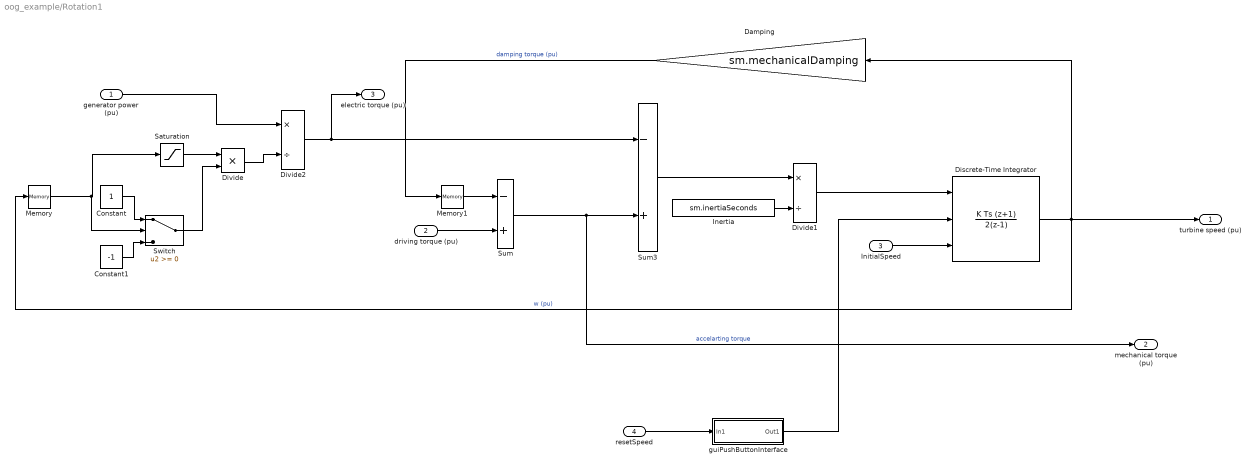
== system oog_example/Rotation1 ==
  generator power (pu) : Inport
  driving torque (pu) : Inport  Port=2
  InitialSpeed : Inport  Port=3
  resetSpeed : Inport  Port=4
  Constant : Constant
  Constant1 : Constant  Value=-1
  Damping : Gain  Gain=sm.mechanicalDamping
  Discrete-Time Integrator : DiscreteIntegrator  IntegratorMethod=Integration: Trapezoidal  ExternalReset=level  InitialConditionSource=external  SampleTime=Ts  LimitOutput=on  UpperSaturationLimit=sm.speedBlockingLimit  LowerSaturationLimit=-sm.speedBlockingLimit  ICPrevOutput=DiscIntNeverNeededParam  ICPrevScaledInput=DiscIntNeverNeededParam
  Divide : Product  Inputs=**
  Divide1 : Product  Inputs=*/
  Divide2 : Product  Inputs=*/
  Inertia : Constant  Value=sm.inertiaSeconds
  Memory : Memory
  Memory1 : Memory
  Saturation : Saturate  UpperLimit=inf  LowerLimit=sm.minSpeedForTorqueCalc
  Sum : Sum  Inputs=-+
  Sum3 : Sum  Inputs=-+
  Switch : Switch
  guiPushButtonInterface : Subsystem
  turbine speed (pu) : Outport
  mechanical torque (pu) : Outport  Port=2
  electric torque (pu) : Outport  Port=3
  wires:
  guiPushButtonInterface/1(Out1) -> Discrete-Time Integrator/2
  resetSpeed/1 -> guiPushButtonInterface/1(In1)
  Constant1/1 -> Switch/3
  Constant/1 -> Switch/1
  Switch/1 -> Divide/2
  Saturation/1 -> Divide/1
  Divide/1 -> Divide2/2
  InitialSpeed/1 -> Discrete-Time Integrator/3
  Discrete-Time Integrator/1 -> Memory/1, turbine speed (pu)/1, Damping/1  "w (pu)"
  Divide1/1 -> Discrete-Time Integrator/1
  Damping/1 -> Memory1/1  "damping torque (pu)"
  Inertia/1 -> Divide1/2
  Sum3/1 -> Divide1/1
  Divide2/1 -> Sum3/1, electric torque (pu)/1
  Sum/1 -> mechanical torque (pu)/1, Sum3/2  "accelarting torque"
  driving torque (pu)/1 -> Sum/2
  generator power (pu)/1 -> Divide2/1
  Memory/1 -> Saturation/1, Switch/2
  Memory1/1 -> Sum/1

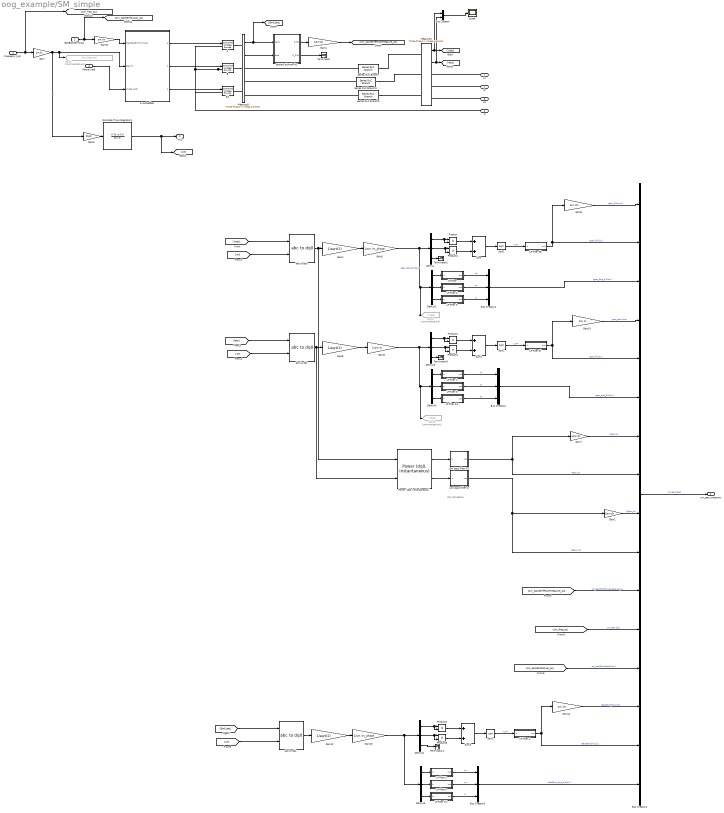
== system oog_example/SM_simple ==
  note: PQ calculation
  Frequency [pu] : Inport
  GenBackEmf [pu] : Inport  Port=2
  Phase [rad] : Inport  Port=3
  A : powerlib/Electrical Sources/Controlled Voltage Source  Initialize=off  Source_Type=DC  Amplitude=0  Phase=0  Frequency=0  Measurements=Voltage
  B : powerlib/Electrical Sources/Controlled Voltage Source  Initialize=off  Source_Type=DC  Amplitude=0  Phase=0  Frequency=0  Measurements=None
  B1 : powerlib/Electrical Sources/Controlled Voltage Source  Initialize=off  Source_Type=DC  Amplitude=0  Phase=0  Frequency=0  Measurements=Voltage
  Bus Creator : BusCreator  Inputs=2
  Bus Creator1 : BusCreator  Inputs=3
  Bus Creator2 : BusCreator  Inputs=3
  Bus Creator3 : BusCreator  Inputs=3
  Bus Creator4 : BusCreator  Inputs=16
  Demux{,1..5} (6 alike) : Demux  Outputs=3
  Discrete-Time Integrator1 : DiscreteIntegrator  IntegratorMethod=Integration: Trapezoidal  SampleTime=Ts  UpperSaturationLimit=sm.speedBlockingLimit  LowerSaturationLimit=-sm.speedBlockingLimit  ICPrevOutput=DiscIntNeverNeededParam  ICPrevScaledInput=DiscIntNeverNeededParam
  Gain : Gain  Gain=sm.fn
  Gain1 : Gain  Gain=1/sm.Sn
  Gain10 : Gain  Gain=sm.In
  Gain11 : Gain  Gain=sm.Vn
  Gain12 : Gain  Gain=1/sqrt(2)
  Gain13 : Gain  Gain=1/sm.Vn_phase
  Gain14 : Gain  Gain=sm.Vn
  Gain2 : Gain  Gain=1/sm.Sn
  Gain3 : Gain  Gain=2*pi()
  Gain4 : Gain  Gain=1/sqrt(2)
  Gain5 : Gain  Gain=1/sm.Vn_phase
  Gain6 : Gain  Gain=sm.Vn
  Gain7 : Gain  Gain=1/sm.Sn
  Gain8 : Gain  Gain=1/sqrt(2)
  Gain9 : Gain  Gain=1/sm.In
  Goto2 : Goto  Commented=on  GotoTag=Vdq0
  Goto5 : Goto  Commented=on  GotoTag=Idq0
  Goto7 : Goto  Commented=on  GotoTag=sm_freq_Hz
  "LP filter " : Subsystem  mask(Discrete first order low pass filter){tau=sm.V_measure_T, Ts=Ts, x0=avr.init, y0=avr.init}
      mask prompts: tau "Filter time constant [s]"; Ts "Sampling time [s]"; x0 "Initial input"; y0 "Initial output"
      mask help: Discrete first order low pass filter derived from a continous filter by bilinear transformation.
  LP filter 1 : Subsystem  mask(Discrete first order low pass filter){tau=sm.I_measure_T, Ts=Ts, x0=0, y0=0}
      mask prompts: tau "Filter time constant [s]"; Ts "Sampling time [s]"; x0 "Initial input"; y0 "Initial output"
      mask help: Discrete first order low pass filter derived from a continous filter by bilinear transformation.
  LP filter 2 : Subsystem  mask(Discrete first order low pass filter){tau=sm.V_measure_T, Ts=Ts, x0=avr.init, y0=avr.init}
      mask prompts: tau "Filter time constant [s]"; Ts "Sampling time [s]"; x0 "Initial input"; y0 "Initial output"
      mask help: Discrete first order low pass filter derived from a continous filter by bilinear transformation.
  LP filter 3 : Subsystem  mask(Discrete first order low pass filter){tau=sm.I_measure_T, Ts=Ts, x0=avr.init, y0=avr.init}
      mask prompts: tau "Filter time constant [s]"; Ts "Sampling time [s]"; x0 "Initial input"; y0 "Initial output"
      mask help: Discrete first order low pass filter derived from a continous filter by bilinear transformation.
  "LP filter 3 " : Subsystem  mask(Discrete first order low pass filter){tau=sm.V_measure_T, Ts=Ts, x0=avr.init, y0=avr.init}
      mask prompts: tau "Filter time constant [s]"; Ts "Sampling time [s]"; x0 "Initial input"; y0 "Initial output"
      mask help: Discrete first order low pass filter derived from a continous filter by bilinear transformation.
  LP filter 3 1 : Subsystem  mask(Discrete first order low pass filter){tau=sm.I_measure_T, Ts=Ts, x0=avr.init, y0=avr.init}
      mask prompts: tau "Filter time constant [s]"; Ts "Sampling time [s]"; x0 "Initial input"; y0 "Initial output"
      mask help: Discrete first order low pass filter derived from a continous filter by bilinear transformation.
  LP filter 3 2 : Subsystem  mask(Discrete first order low pass filter){tau=sm.V_measure_T, Ts=Ts, x0=avr.init, y0=avr.init}
      mask prompts: tau "Filter time constant [s]"; Ts "Sampling time [s]"; x0 "Initial input"; y0 "Initial output"
      mask help: Discrete first order low pass filter derived from a continous filter by bilinear transformation.
  LP filter 4 : Subsystem  mask(Discrete first order low pass filter){tau=sm.V_measure_T, Ts=Ts, x0=avr.init, y0=avr.init}
      mask prompts: tau "Filter time constant [s]"; Ts "Sampling time [s]"; x0 "Initial input"; y0 "Initial output"
      mask help: Discrete first order low pass filter derived from a continous filter by bilinear transformation.
  LP filter 5 : Subsystem  mask(Discrete first order low pass filter){tau=sm.V_measure_T, Ts=Ts, x0=avr.init, y0=avr.init}
      mask prompts: tau "Filter time constant [s]"; Ts "Sampling time [s]"; x0 "Initial input"; y0 "Initial output"
      mask help: Discrete first order low pass filter derived from a continous filter by bilinear transformation.
  LP filter 6 : Subsystem  mask(Discrete first order low pass filter){tau=sm.V_measure_T, Ts=Ts, x0=avr.init, y0=avr.init}
      mask prompts: tau "Filter time constant [s]"; Ts "Sampling time [s]"; x0 "Initial input"; y0 "Initial output"
      mask help: Discrete first order low pass filter derived from a continous filter by bilinear transformation.
  LP filter 66 : Subsystem  mask(Discrete first order low pass filter){tau=sm.V_measure_T, Ts=Ts, x0=avr.init, y0=avr.init}
      mask prompts: tau "Filter time constant [s]"; Ts "Sampling time [s]"; x0 "Initial input"; y0 "Initial output"
      mask help: Discrete first order low pass filter derived from a continous filter by bilinear transformation.
  LP filter 67 : Subsystem  mask(Discrete first order low pass filter){tau=sm.I_measure_T, Ts=Ts, x0=avr.init, y0=avr.init}
      mask prompts: tau "Filter time constant [s]"; Ts "Sampling time [s]"; x0 "Initial input"; y0 "Initial output"
      mask help: Discrete first order low pass filter derived from a continous filter by bilinear transformation.
  Low pass filter P1 : Subsystem  mask(Discrete first order low pass filter){tau=sm.P_measure, Ts=Ts, x0=0, y0=0}
      mask prompts: tau "Filter time constant [s]"; Ts "Sampling time [s]"; x0 "Initial input"; y0 "Initial output"
      mask help: Discrete first order low pass filter derived from a continous filter by bilinear transformation.
  Low pass filter Q : Subsystem  mask(Discrete first order low pass filter){tau=sm.Q_measure, Ts=Ts, x0=0, y0=0}
      mask prompts: tau "Filter time constant [s]"; Ts "Sampling time [s]"; x0 "Initial input"; y0 "Initial output"
      mask help: Discrete first order low pass filter derived from a continous filter by bilinear transformation.
  Measure1 : powerlib/Measurements/Three-Phase V-I Measurement  VoltageMeasurement=phase-to-ground  SetLabelV=off  LabelV=genOut  Vpu=off  VpuLL=off  CurrentMeasurement=yes  SetLabelI=off  LabelI=genCurrentOut  Ipu=off  Pbase=1e3  Vbase=380  OutputType=Magnitude  PhasorSimulation=off  PSBequivalent=0
  Measure3 : powerlib/Measurements/Three-Phase V-I Measurement  VoltageMeasurement=phase-to-ground  SetLabelV=off  LabelV=genOut  Vpu=off  VpuLL=off  CurrentMeasurement=yes  SetLabelI=off  LabelI=genCurrentOut  Ipu=off  Pbase=1e3  Vbase=380  OutputType=Magnitude  PhasorSimulation=off  PSBequivalent=0
  "Power (dq0, Instantaneous)" : powerlib_meascontrol/Measurements/Power (dq0, Instantaneous)
  Product{,1..5} (6 alike) : Product
  Scope : Scope
  Series RLC Branch : powerlib/Elements/Series RLC Branch  LConnTagsString=__new0  RConnTagsString=__new0  BranchType=RL  Resistance=sm.R  Inductance=sm.L  SetiL0=off  InitialCurrent=0  Capacitance=1e-6  Setx0=off  InitialVoltage=0  Measurements=None
  Series RLC Branch1 : powerlib/Elements/Series RLC Branch  LConnTagsString=__new0  RConnTagsString=__new0  BranchType=RL  Resistance=sm.R  Inductance=sm.L  SetiL0=off  InitialCurrent=0  Capacitance=1e-6  Setx0=off  InitialVoltage=0  Measurements=None
  Series RLC Branch2 : powerlib/Elements/Series RLC Branch  LConnTagsString=__new0  RConnTagsString=__new0  BranchType=RL  Resistance=sm.R  Inductance=sm.L  SetiL0=off  InitialCurrent=0  Capacitance=1e-6  Setx0=off  InitialVoltage=0  Measurements=None
  Sqrt1 : Sqrt  SaturateOnIntegerOverflow=on
  Sqrt2 : Sqrt  SaturateOnIntegerOverflow=on
  Sqrt3 : Sqrt  SaturateOnIntegerOverflow=on
  Sum : Sum
  Sum1 : Sum
  Sum2 : Sum
  Terminator{,1..3} (4 alike) : Terminator
  abc to dq0 : powerlib_meascontrol/Transformations/abc to dq0  Alignment=Aligned with phase A axis
  abc to dq1 : powerlib_meascontrol/Transformations/abc to dq0  Alignment=Aligned with phase A axis
  abc to dq2 : powerlib_meascontrol/Transformations/abc to dq0  Alignment=Aligned with phase A axis
  powerCalcAndFilt1 : Subsystem
  sinusRefGen : Subsystem
  L1 : PMIOPort  Port=1  Side=Right
  L2 : PMIOPort  Port=2  Side=Right
  L3 : PMIOPort  Port=3  Side=Right
  N : PMIOPort  Port=4  Side=Right
  wt1 : Outport
  sm_gen_measure : Outport  Port=2
  wires:
  abc to dq1/1 -> Gain8/1, "Power (dq0, Instantaneous)"/2
  Gain13/1 -> Demux2/1, Demux5/1
  LP filter 3 2/1(out) -> Bus Creator3/3  "0"
  LP filter 6/1(out) -> Bus Creator3/2  "vq"
  LP filter 5/1(out) -> Bus Creator3/1  "vd"
  Bus Creator3/1 -> Bus Creator4/16  "BackEmf_dqo_filt [pu]"
  Demux5/1 -> LP filter 5/1(in)
  Demux5/3 -> LP filter 3 2/1(in)
  Demux5/2 -> LP filter 6/1(in)
  Gain14/1 -> Bus Creator4/14  "BackEmf_filt [rms]"
  [wt] -> abc to dq2/2
  LP filter 4/1(out) -> Bus Creator4/15, Gain14/1  "BackEmf_filt [pu]"
  Sqrt3/1 -> LP filter 4/1(in)  "v_pu"
  Sum2/1 -> Sqrt3/1
  Product5/1 -> Sum2/2
  Demux2/2 -> Product5/1, Product5/2
  Product4/1 -> Sum2/1
  Demux2/1 -> Product4/1, Product4/2
  [Emf_abc] -> abc to dq2/1
  Gain12/1 -> Gain13/1
  abc to dq2/1 -> Gain12/1
  Frequency [pu]/1 -> Gain/1, [sm_freq_pu]
  [sm_backEmfActual_pu] -> Bus Creator4/13  "sm_backEmfActual [pu]"
  [sm_freq_pu] -> Bus Creator4/12  "sm_freq [pu]"
  Gain11/1 -> sinusRefGen/1(GenBackEmf [VrmsLL])
  [sm_backEmfPowerMeasure_pu] -> Bus Creator4/11  "sm_backEmfPowerMeasure_pu"
  Bus Creator4/1 -> sm_gen_measure/1  "sm_genMeas"
  Low pass filter Q/1(out) -> Gain2/1, Bus Creator4/10  "Qgen_VAr"
  Low pass filter P1/1(out) -> Gain7/1, Bus Creator4/8  "Pgen_W"
  "Power (dq0, Instantaneous)"/2 -> Low pass filter Q/1(in)
  "Power (dq0, Instantaneous)"/1 -> Low pass filter P1/1(in)
  Bus Creator/1 -> Scope/1
  Gain5/1 -> Demux/1, Demux1/1, Goto2/1  "Vgen_dqo_filt [pu]"
  Gain10/1 -> Bus Creator4/4  "Igen_abc [rms]"
  LP filter 3 1/1(out) -> Bus Creator2/3  "I0"
  LP filter 3/1(out) -> Bus Creator2/2  "Iq"
  LP filter 1/1(out) -> Bus Creator2/1  "Id"
  Bus Creator2/1 -> Bus Creator4/6  "Igen_dqo_filt [pu]"
  Demux4/1 -> LP filter 1/1(in)
  Demux4/3 -> LP filter 3 1/1(in)
  Demux4/2 -> LP filter 3/1(in)
  [wt] -> abc to dq1/2
  LP filter 67/1(out) -> Bus Creator4/5, Gain10/1  "Igen_filt [pu]"
  Sqrt2/1 -> LP filter 67/1(in)  "v_pu"
  Sum1/1 -> Sqrt2/1
  Product3/1 -> Sum1/2
  Demux3/2 -> Product3/1, Product3/2
  Product2/1 -> Sum1/1
  Demux3/1 -> Product2/1, Product2/2
  Gain9/1 -> Demux3/1, Demux4/1, Goto5/1
  [Iabc] -> abc to dq1/1
  Gain8/1 -> Gain9/1
  Measure1/2 -> [Iabc], Bus Creator/2
  Gain6/1 -> Bus Creator4/1  "Vgen_filt [rms]"
  Measure1/1 -> [Vabc], Bus Creator/1
  "LP filter 3 "/1(out) -> Bus Creator1/3  "0"
  LP filter 2/1(out) -> Bus Creator1/2  "vq"
  "LP filter "/1(out) -> Bus Creator1/1  "vd"
  Bus Creator1/1 -> Bus Creator4/3  "Vgen_dqo_filt [pu]"
  Demux1/1 -> "LP filter "/1(in)
  Demux1/3 -> "LP filter 3 "/1(in)
  Demux1/2 -> LP filter 2/1(in)
  [wt] -> abc to dq0/2
  powerCalcAndFilt1/2(Q_filt1) -> Terminator/1
  Gain1/1 -> [sm_backEmfPowerMeasure_pu]
  powerCalcAndFilt1/1(P_filt) -> Gain1/1
  Measure3/2 -> powerCalcAndFilt1/2(Iabc)
  Measure3/1 -> powerCalcAndFilt1/1(Vabc), [Emf_abc]
  LP filter 66/1(out) -> Bus Creator4/2, Gain6/1  "Vgen_filt [pu]"
  Sqrt1/1 -> LP filter 66/1(in)  "v_pu"
  Sum/1 -> Sqrt1/1
  Product1/1 -> Sum/2
  Demux/2 -> Product1/1, Product1/2
  Product/1 -> Sum/1
  Demux/1 -> Product/1, Product/2
  [Vabc] -> abc to dq0/1
  Gain4/1 -> Gain5/1
  Gain3/1 -> Discrete-Time Integrator1/1
  Gain/1 -> Goto7/1, sinusRefGen/2(freq Hz), Gain3/1  "f"
  abc to dq0/1 -> Gain4/1, "Power (dq0, Instantaneous)"/1
  Discrete-Time Integrator1/1 -> wt1/1, [wt]
  Gain2/1 -> Bus Creator4/9  "Qgen_pu"
  Gain7/1 -> Bus Creator4/7  "Pgen_pu"
  sinusRefGen/3(c) -> B1/1
  sinusRefGen/2(b) -> B/1
  sinusRefGen/1(a) -> A/1
  Phase [rad]/1 -> sinusRefGen/3(phase (rad))
  GenBackEmf [pu]/1 -> Gain11/1, [sm_backEmfActual_pu]
  Demux2/3 -> Terminator1/1
  Demux/3 -> Terminator2/1
  Demux3/3 -> Terminator3/1
  connections:
  Series RLC Branch/LConn1 -- Measure3/RConn1
  Series RLC Branch1/LConn1 -- Measure3/RConn2
  Series RLC Branch2/LConn1 -- Measure3/RConn3
  L1/RConn1 -- Measure1/RConn1
  L2/RConn1 -- Measure1/RConn2
  L3/RConn1 -- Measure1/RConn3
  Series RLC Branch2/RConn1 -- Measure1/LConn3
  Series RLC Branch1/RConn1 -- Measure1/LConn2
  Series RLC Branch/RConn1 -- Measure1/LConn1
  Measure3/LConn3 -- B1/RConn1
  Measure3/LConn2 -- B/RConn1
  A/RConn1 -- Measure3/LConn1
  B/LConn1 -- B1/LConn1 -- N/RConn1 -- A/LConn1
